simulink model "three_phase_inverter"  (R2014a)
settings: Solver=ode45  StartTime=0.0  StopTime=0.06  MaxStep=0.001  RelTol=1e-3
libraries: powerlib x33
settings Model: Creator=User  LastModifiedBy=User

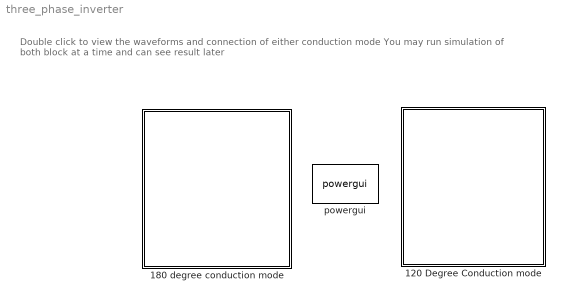
== system three_phase_inverter ==
  note: Double click to view the waveforms and connection of either conduction mode
      | You may run simulation of both block at a time and can see result later
  120 Degree Conduction mode : Subsystem
      mask Display: fprintf('120 degree \n conduction mode')
  180 degree conduction mode : Subsystem
      mask Display: fprintf('180 degree \n conduction mode')
  powergui : powerlib/powergui  Priority=1  SimulationMode=Continuous  SolverType=Tustin  SampleTime=50e-6  frequency=60  SPID=off  DisableSnubberDevices=off  DisableRonSwitches=off  DisableVfSwitches=off  SwTol=0  Interpol=off  DisplayEquations=off  Ts=0  methode=off  frequencyindice=0  Pbase=100e6  ErrMax=1e-4  Iterations=50  UnitsV=kV  UnitsW=MW  FunctionMessages=off  echomessages=off  HookPort=off  EnableUseOfTLC=off  x0status=blocks  RestoreLinks=warning  ResistiveCurrentMeasurement=off  Frange=[0:2:500]  Ylog=off  Xlog=on  ShowGrid=off  save=off  variable=ZData  structure=0  ZoomFFT=off  StartTime=0.0  cycles=1  DisplayStyle=1  fundamental=60  FreqAxis=off  MaxFrequency=1000  frequencyindicesteady=1  RmsSteady=1  display=off

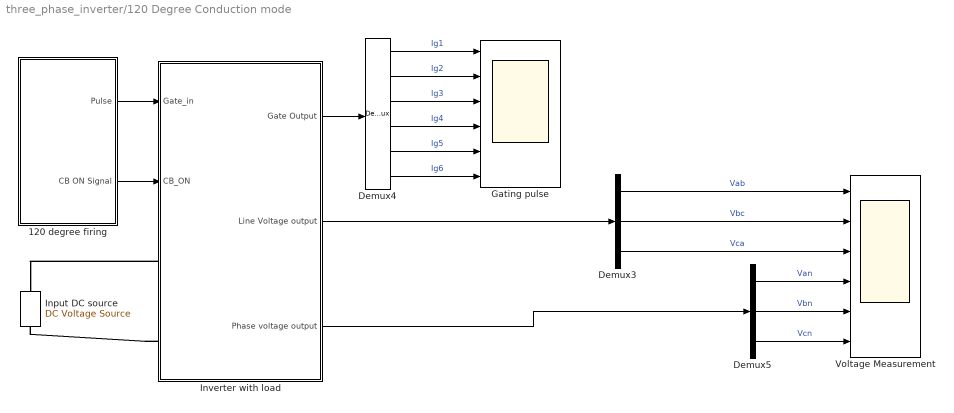
== system three_phase_inverter/120 Degree Conduction mode ==
  120 degree firing : Subsystem  mask{f=50, t=0}
      mask prompts: f "Enter required output frequency"; t "Enter Inverter On time in seconds"
  Demux3 : Demux  Outputs=3
  Demux4 : Demux  Outputs=6
  Demux5 : Demux  Outputs=3
  Gating pulse : Scope  NumInputPorts=6
      settings: ShowLegends=on  YMin=-5~-5~-5~-5~-5~-5  YMax=5~5~5~5~5~5  SaveName=ScopeData2
  Input DC source : powerlib/Electrical Sources/DC Voltage Source  Amplitude=400  Measurements=None
  Inverter with load : Subsystem
  Voltage Measurement : Scope  NumInputPorts=6
      settings: ShowLegends=on  YMin=-5~-5~-5~-5~-5~-5  YMax=5~5~5~5~5~5  SaveName=ScopeData3
  wires:
  Demux4/6 -> Gating pulse/6  "Ig6"
  Inverter with load/2(Line Voltage output) -> Demux3/1
  Demux4/5 -> Gating pulse/5  "Ig5"
  Demux4/2 -> Gating pulse/2  "Ig2"
  Demux3/1 -> Voltage Measurement/1  "Vab"
  120 degree firing/2(CB ON Signal) -> Inverter with load/2(CB_ON)
  Demux4/1 -> Gating pulse/1  "Ig1"
  Demux5/2 -> Voltage Measurement/5  "Vbn"
  Demux4/3 -> Gating pulse/3  "Ig3"
  Demux5/3 -> Voltage Measurement/6  "Vcn"
  Demux5/1 -> Voltage Measurement/4  "Van"
  Demux3/2 -> Voltage Measurement/2  "Vbc"
  Inverter with load/1(Gate Output) -> Demux4/1
  120 degree firing/1(Pulse) -> Inverter with load/1(Gate_in)
  Demux3/3 -> Voltage Measurement/3  "Vca"
  Demux4/4 -> Gating pulse/4  "Ig4"
  Inverter with load/3(Phase voltage output) -> Demux5/1
  connections:
  Inverter with load/LConn1 -- Input DC source/RConn1
  Inverter with load/LConn2 -- Input DC source/LConn1

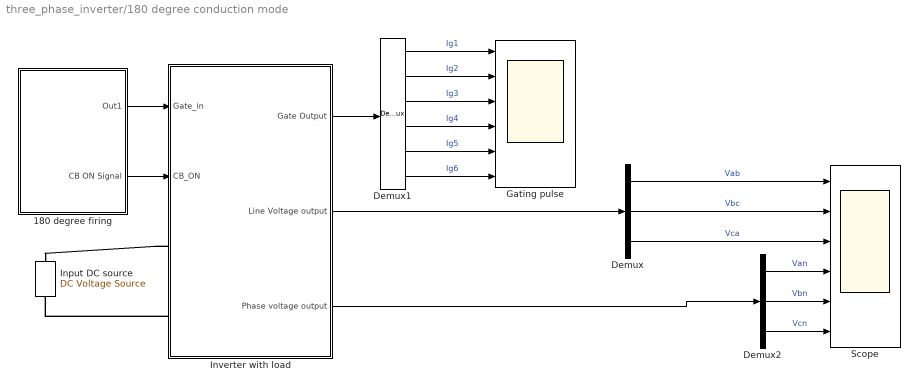
== system three_phase_inverter/180 degree conduction mode ==
  180 degree firing : Subsystem  mask{f=50, t=0}
      mask prompts: f "Enter required output frequency"; t "Enter time to turn ON circuit Breaker in seconds"
  Demux : Demux  Outputs=3
  Demux1 : Demux  Outputs=6
  Demux2 : Demux  Outputs=3
  Gating pulse : Scope  NumInputPorts=6
      settings: ShowLegends=on  YMin=-5~-5~-5~-5~-5~-5  YMax=5~5~5~5~5~5
  Input DC source : powerlib/Electrical Sources/DC Voltage Source  Amplitude=400  Measurements=None
  Inverter with load : Subsystem
  Scope : Scope  NumInputPorts=6
      settings: ShowLegends=on  YMin=-5~-5~-5~-5~-5~-5  YMax=5~5~5~5~5~5
  wires:
  Demux/1 -> Scope/1  "Vab"
  Demux/2 -> Scope/2  "Vbc"
  Demux2/1 -> Scope/4  "Van"
  Demux2/2 -> Scope/5  "Vbn"
  Demux1/4 -> Gating pulse/4  "Ig4"
  Inverter with load/3(Phase voltage output) -> Demux2/1
  Demux1/3 -> Gating pulse/3  "Ig3"
  180 degree firing/1(Out1) -> Inverter with load/1(Gate_in)
  Demux1/6 -> Gating pulse/6  "Ig6"
  Demux1/2 -> Gating pulse/2  "Ig2"
  Demux/3 -> Scope/3  "Vca"
  Demux1/5 -> Gating pulse/5  "Ig5"
  Demux1/1 -> Gating pulse/1  "Ig1"
  Demux2/3 -> Scope/6  "Vcn"
  Inverter with load/1(Gate Output) -> Demux1/1
  Inverter with load/2(Line Voltage output) -> Demux/1
  180 degree firing/2(CB ON Signal) -> Inverter with load/2(CB_ON)
  connections:
  Inverter with load/LConn2 -- Input DC source/LConn1
  Inverter with load/LConn1 -- Input DC source/RConn1

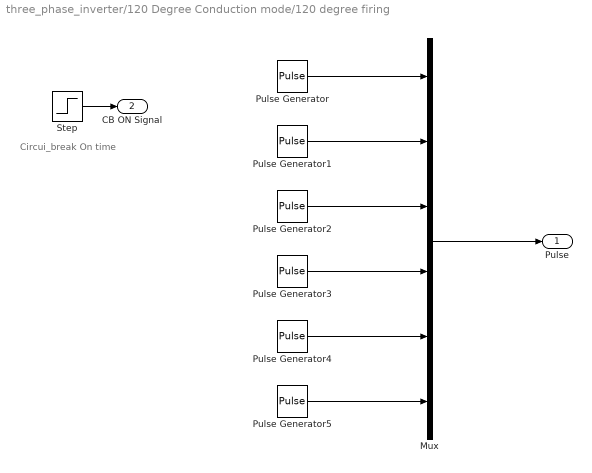
== system three_phase_inverter/120 Degree Conduction mode/120 degree firing ==
  note: Circui_break On time
  Mux : Mux  Inputs=6
  Pulse Generator : DiscretePulseGenerator  PulseType=Time based  Amplitude=5  Period=1/f  PulseWidth=(120/360)*100
  Pulse Generator1 : DiscretePulseGenerator  PulseType=Time based  Amplitude=5  Period=1/f  PulseWidth=(120/360)*100  PhaseDelay=(0.01*60/180)
  Pulse Generator2 : DiscretePulseGenerator  PulseType=Time based  Amplitude=5  Period=1/f  PulseWidth=(120/360)*100  PhaseDelay=0.01*120/180
  Pulse Generator3 : DiscretePulseGenerator  PulseType=Time based  Amplitude=5  Period=1/f  PulseWidth=(120/360)*100  PhaseDelay=0.01
  Pulse Generator4 : DiscretePulseGenerator  PulseType=Time based  Amplitude=5  Period=1/f  PulseWidth=(120/360)*100  PhaseDelay=0.01*240/180
  Pulse Generator5 : DiscretePulseGenerator  PulseType=Time based  Amplitude=5  Period=1/f  PulseWidth=(120/360)*100  PhaseDelay=-0.01*60/180
  Step : Step  Time=t  SampleTime=0
  Pulse : Outport
  CB ON Signal : Outport  Port=2
  wires:
  Pulse Generator/1 -> Mux/1
  Mux/1 -> Pulse/1
  Pulse Generator2/1 -> Mux/3
  Pulse Generator1/1 -> Mux/2
  Pulse Generator3/1 -> Mux/4
  Pulse Generator4/1 -> Mux/5
  Pulse Generator5/1 -> Mux/6
  Step/1 -> CB ON Signal/1

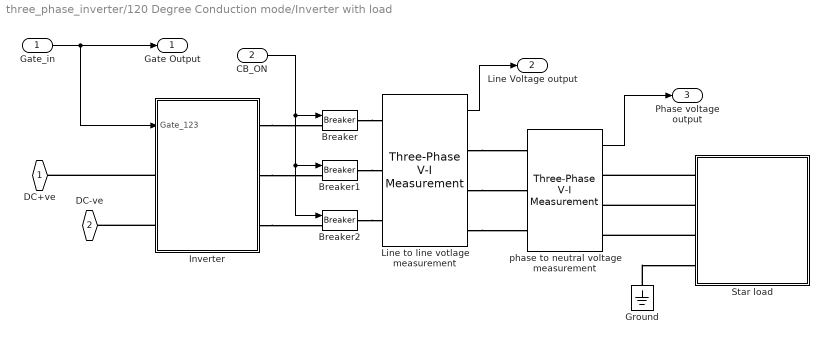
== system three_phase_inverter/120 Degree Conduction mode/Inverter with load ==
  Gate_in : Inport
  CB_ON : Inport  Port=2
  Breaker : powerlib/Elements/Breaker  InitialState=0  SwitchingTimes="[1/60  5/60]"  External=on  BreakerResistance=0.01  SnubberResistance=1e6  SnubberCapacitance=inf  Measurements=None  MoreParameters=on  NoBreakLoop=off
  Breaker1 : powerlib/Elements/Breaker  InitialState=0  SwitchingTimes="[1/60  5/60]"  External=on  BreakerResistance=0.01  SnubberResistance=1e6  SnubberCapacitance=inf  Measurements=None  MoreParameters=on  NoBreakLoop=off
  Breaker2 : powerlib/Elements/Breaker  InitialState=0  SwitchingTimes="[1/60  5/60]"  External=on  BreakerResistance=0.01  SnubberResistance=1e6  SnubberCapacitance=inf  Measurements=None  MoreParameters=on  NoBreakLoop=off
  Ground : powerlib/Elements/Ground  LConnTagsString=a
  Inverter : Subsystem
  Line to line votlage measurement : powerlib/Measurements/Three-Phase V-I Measurement  VoltageMeasurement=phase-to-phase  SetLabelV=off  LabelV=Vabc  Vpu=off  VpuLL=off  CurrentMeasurement=no  SetLabelI=off  LabelI=Iabc  Ipu=off  Pbase=100e6  Vbase=500e3  OutputType=Complex  PhasorSimulation=off  PSBequivalent=0
  Star load : Subsystem
  phase to neutral voltage measurement : powerlib/Measurements/Three-Phase V-I Measurement  VoltageMeasurement=phase-to-ground  SetLabelV=off  LabelV=Vabc  Vpu=off  VpuLL=off  CurrentMeasurement=no  SetLabelI=off  LabelI=Iabc  Ipu=off  Pbase=100e6  Vbase=500e3  OutputType=Complex  PhasorSimulation=off  PSBequivalent=0
  DC+ve : PMIOPort  Port=1  Side=Left
  DC-ve : PMIOPort  Port=2  Side=Left
  Gate Output : Outport
  Line Voltage output : Outport  Port=2
  Phase voltage output : Outport  Port=3
  wires:
  phase to neutral voltage measurement/1 -> Phase voltage output/1
  Line to line votlage measurement/1 -> Line Voltage output/1
  Gate_in/1 -> Gate Output/1, Inverter/1(Gate_123)
  CB_ON/1 -> Breaker2/1, Breaker1/1, Breaker/1
  connections:
  Ground/LConn1 -- Star load/LConn4
  Star load/LConn2 -- phase to neutral voltage measurement/RConn2
  Star load/LConn1 -- phase to neutral voltage measurement/RConn1
  Line to line votlage measurement/RConn3 -- phase to neutral voltage measurement/LConn3
  Line to line votlage measurement/RConn2 -- phase to neutral voltage measurement/LConn2
  Inverter/LConn2 -- DC-ve/RConn1
  Line to line votlage measurement/RConn1 -- phase to neutral voltage measurement/LConn1
  Inverter/LConn1 -- DC+ve/RConn1
  Star load/LConn3 -- phase to neutral voltage measurement/RConn3
  Inverter/RConn1 -- Breaker/LConn1
  Breaker/RConn1 -- Line to line votlage measurement/LConn1
  Inverter/RConn3 -- Breaker2/LConn1
  Inverter/RConn2 -- Breaker1/LConn1
  Breaker1/RConn1 -- Line to line votlage measurement/LConn2
  Breaker2/RConn1 -- Line to line votlage measurement/LConn3

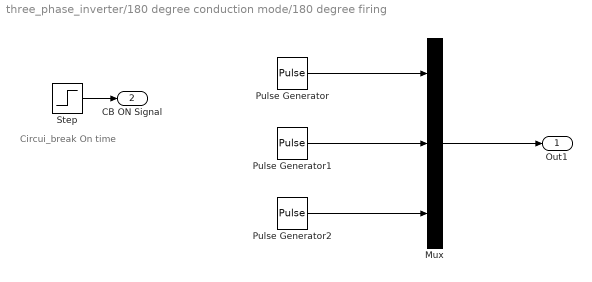
== system three_phase_inverter/180 degree conduction mode/180 degree firing ==
  note: Circui_break On time
  Mux : Mux  Inputs=3
  Pulse Generator : DiscretePulseGenerator  PulseType=Time based  Amplitude=5  Period=1/f  PulseWidth=50
  Pulse Generator1 : DiscretePulseGenerator  PulseType=Time based  Amplitude=5  Period=1/f  PulseWidth=50  PhaseDelay=(0.01*60/180)
  Pulse Generator2 : DiscretePulseGenerator  PulseType=Time based  Amplitude=5  Period=1/f  PulseWidth=50  PhaseDelay=0.01*120/180
  Step : Step  Time=t  SampleTime=0
  Out1 : Outport
  CB ON Signal : Outport  Port=2
  wires:
  Pulse Generator1/1 -> Mux/2
  Pulse Generator2/1 -> Mux/3
  Mux/1 -> Out1/1
  Pulse Generator/1 -> Mux/1
  Step/1 -> CB ON Signal/1

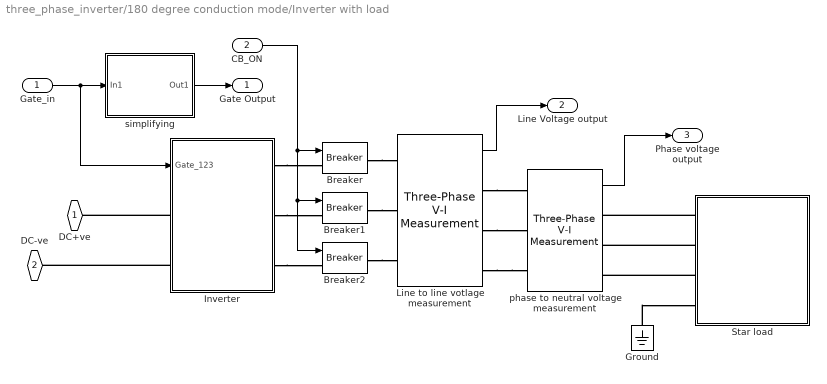
== system three_phase_inverter/180 degree conduction mode/Inverter with load ==
  Gate_in : Inport
  CB_ON : Inport  Port=2
  Breaker : powerlib/Elements/Breaker  InitialState=0  SwitchingTimes="[1/60  5/60]"  External=on  BreakerResistance=0.01  SnubberResistance=1e6  SnubberCapacitance=inf  Measurements=None  MoreParameters=on  NoBreakLoop=off
  Breaker1 : powerlib/Elements/Breaker  InitialState=0  SwitchingTimes="[1/60  5/60]"  External=on  BreakerResistance=0.01  SnubberResistance=1e6  SnubberCapacitance=inf  Measurements=None  MoreParameters=on  NoBreakLoop=off
  Breaker2 : powerlib/Elements/Breaker  InitialState=0  SwitchingTimes="[1/60  5/60]"  External=on  BreakerResistance=0.01  SnubberResistance=1e6  SnubberCapacitance=inf  Measurements=None  MoreParameters=on  NoBreakLoop=off
  Ground : powerlib/Elements/Ground  LConnTagsString=a
  Inverter : Subsystem
  Line to line votlage measurement : powerlib/Measurements/Three-Phase V-I Measurement  VoltageMeasurement=phase-to-phase  SetLabelV=off  LabelV=Vabc  Vpu=off  VpuLL=off  CurrentMeasurement=no  SetLabelI=off  LabelI=Iabc  Ipu=off  Pbase=100e6  Vbase=500e3  OutputType=Complex  PhasorSimulation=off  PSBequivalent=0
  Star load : Subsystem
  phase to neutral voltage measurement : powerlib/Measurements/Three-Phase V-I Measurement  VoltageMeasurement=phase-to-ground  SetLabelV=off  LabelV=Vabc  Vpu=off  VpuLL=off  CurrentMeasurement=no  SetLabelI=off  LabelI=Iabc  Ipu=off  Pbase=100e6  Vbase=500e3  OutputType=Complex  PhasorSimulation=off  PSBequivalent=0
  simplifying : Subsystem
  DC+ve : PMIOPort  Port=1  Side=Left
  DC-ve : PMIOPort  Port=2  Side=Left
  Gate Output : Outport
  Line Voltage output : Outport  Port=2
  Phase voltage output : Outport  Port=3
  wires:
  simplifying/1(Out1) -> Gate Output/1
  Line to line votlage measurement/1 -> Line Voltage output/1
  Gate_in/1 -> Inverter/1(Gate_123), simplifying/1(In1)
  phase to neutral voltage measurement/1 -> Phase voltage output/1
  CB_ON/1 -> Breaker2/1, Breaker1/1, Breaker/1
  connections:
  Star load/LConn3 -- phase to neutral voltage measurement/RConn3
  Inverter/LConn1 -- DC+ve/RConn1
  Line to line votlage measurement/RConn1 -- phase to neutral voltage measurement/LConn1
  Inverter/LConn2 -- DC-ve/RConn1
  Line to line votlage measurement/RConn2 -- phase to neutral voltage measurement/LConn2
  Line to line votlage measurement/RConn3 -- phase to neutral voltage measurement/LConn3
  Star load/LConn1 -- phase to neutral voltage measurement/RConn1
  Star load/LConn2 -- phase to neutral voltage measurement/RConn2
  Ground/LConn1 -- Star load/LConn4
  Inverter/RConn1 -- Breaker/LConn1
  Inverter/RConn2 -- Breaker1/LConn1
  Inverter/RConn3 -- Breaker2/LConn1
  Breaker/RConn1 -- Line to line votlage measurement/LConn1
  Breaker1/RConn1 -- Line to line votlage measurement/LConn2
  Breaker2/RConn1 -- Line to line votlage measurement/LConn3

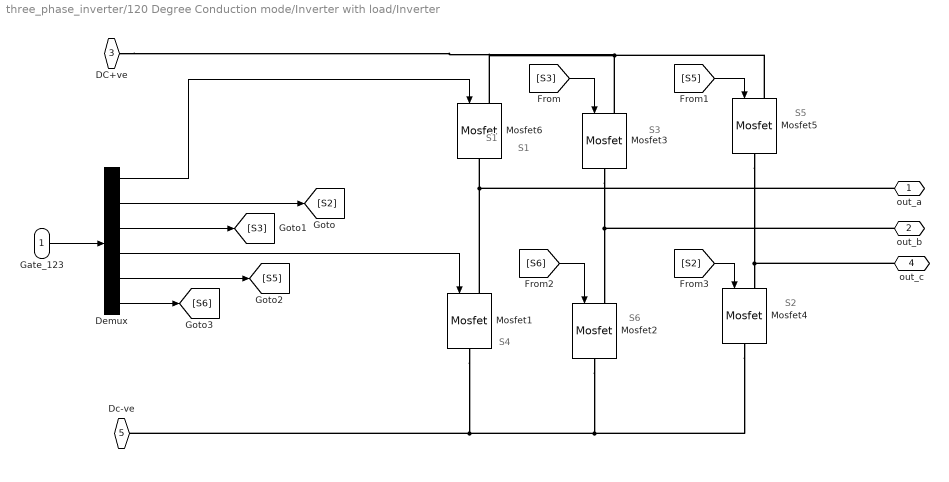
== system three_phase_inverter/120 Degree Conduction mode/Inverter with load/Inverter ==
  note: S1
  note: S3
  note: S5
  note: S2
  note: S4
  note: S6
  note: S1
  Gate_123 : Inport
  Demux : Demux  Outputs=6
  Mosfet{1..6} (6 alike) : powerlib/Power Electronics/Mosfet  Ron=0.1  Lon=0  Rd=0.01  Vfd=0  IC=0  Rs=1e5  Cs=inf  Measurements=off
  out_a : PMIOPort  Port=1  Side=Right
  out_b : PMIOPort  Port=2  Side=Right
  DC+ve : PMIOPort  Port=3  Side=Left
  out_c : PMIOPort  Port=4  Side=Right
  Dc-ve : PMIOPort  Port=5  Side=Left
  wires:
  [S5] -> Mosfet5/1
  [S2] -> Mosfet4/1
  [S6] -> Mosfet2/1
  [S3] -> Mosfet3/1
  Demux/1 -> Mosfet6/1
  Gate_123/1 -> Demux/1
  Demux/2 -> [S2]
  Demux/3 -> [S3]
  Demux/4 -> Mosfet1/1
  Demux/5 -> [S5]
  Demux/6 -> [S6]
  connections:
  out_c/RConn1 -- Mosfet5/RConn1 -- Mosfet4/LConn1
  out_b/RConn1 -- Mosfet2/LConn1 -- Mosfet3/RConn1
  Mosfet4/RConn1 -- Mosfet2/RConn1 -- Mosfet1/RConn1 -- Dc-ve/RConn1
  Mosfet5/LConn1 -- Mosfet6/LConn1 -- DC+ve/RConn1 -- Mosfet3/LConn1
  out_a/RConn1 -- Mosfet1/LConn1 -- Mosfet6/RConn1

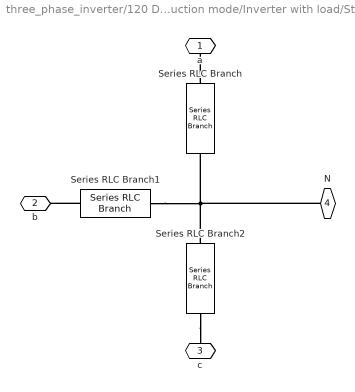
== system three_phase_inverter/120 Degree Conduction mode/Inverter with load/Star load ==
  Series RLC Branch : powerlib/Elements/Series RLC Branch  LConnTagsString=__new0  RConnTagsString=__new0  BranchType=R  Resistance=10  Inductance=1e-3  SetiL0=off  InitialCurrent=0  Capacitance=1e-6  Setx0=off  InitialVoltage=0  Measurements=None
  Series RLC Branch1 : powerlib/Elements/Series RLC Branch  LConnTagsString=__new0  RConnTagsString=__new0  BranchType=R  Resistance=10  Inductance=1e-3  SetiL0=off  InitialCurrent=0  Capacitance=1e-6  Setx0=off  InitialVoltage=0  Measurements=None
  Series RLC Branch2 : powerlib/Elements/Series RLC Branch  LConnTagsString=__new0  RConnTagsString=__new0  BranchType=R  Resistance=10  Inductance=1e-3  SetiL0=off  InitialCurrent=0  Capacitance=1e-6  Setx0=off  InitialVoltage=0  Measurements=None
  a : PMIOPort  Port=1  Side=Left
  b : PMIOPort  Port=2  Side=Left
  c : PMIOPort  Port=3  Side=Left
  N : PMIOPort  Port=4  Side=Left
  connections:
  Series RLC Branch/LConn1 -- a/RConn1
  Series RLC Branch1/RConn1 -- b/RConn1
  Series RLC Branch2/RConn1 -- c/RConn1
  Series RLC Branch2/LConn1 -- N/RConn1 -- Series RLC Branch/RConn1 -- Series RLC Branch1/LConn1

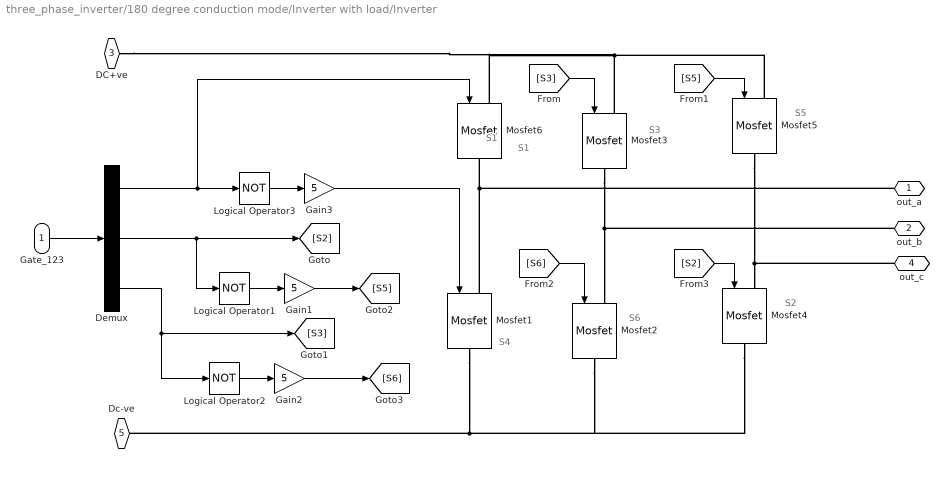
== system three_phase_inverter/180 degree conduction mode/Inverter with load/Inverter ==
  note: S1
  note: S6
  note: S4
  note: S2
  note: S5
  note: S3
  note: S1
  Gate_123 : Inport
  Demux : Demux  Outputs=3
  Gain1 : Gain  Gain=5
  Gain2 : Gain  Gain=5
  Gain3 : Gain  Gain=5
  Logical Operator1 : Logic  Operator=NOT  AllPortsSameDT=off  OutDataTypeStr=boolean
  Logical Operator2 : Logic  Operator=NOT  AllPortsSameDT=off  OutDataTypeStr=boolean
  Logical Operator3 : Logic  Operator=NOT  AllPortsSameDT=off  OutDataTypeStr=boolean
  Mosfet{1..6} (6 alike) : powerlib/Power Electronics/Mosfet  Ron=0.1  Lon=0  Rd=0.01  Vfd=0  IC=0  Rs=1e5  Cs=inf  Measurements=off
  out_a : PMIOPort  Port=1  Side=Right
  out_b : PMIOPort  Port=2  Side=Right
  DC+ve : PMIOPort  Port=3  Side=Left
  out_c : PMIOPort  Port=4  Side=Right
  Dc-ve : PMIOPort  Port=5  Side=Left
  wires:
  Gate_123/1 -> Demux/1
  Logical Operator3/1 -> Gain3/1
  Demux/1 -> Logical Operator3/1, Mosfet6/1
  Gain3/1 -> Mosfet1/1
  Demux/2 -> Logical Operator1/1, [S2]
  Demux/3 -> [S3], Logical Operator2/1
  Logical Operator1/1 -> Gain1/1
  Logical Operator2/1 -> Gain2/1
  Gain1/1 -> [S5]
  Gain2/1 -> [S6]
  [S3] -> Mosfet3/1
  [S6] -> Mosfet2/1
  [S2] -> Mosfet4/1
  [S5] -> Mosfet5/1
  connections:
  Mosfet1/LConn1 -- out_a/RConn1 -- Mosfet6/RConn1
  DC+ve/RConn1 -- Mosfet6/LConn1 -- Mosfet5/LConn1 -- Mosfet3/LConn1
  Mosfet1/RConn1 -- Mosfet4/RConn1 -- Mosfet2/RConn1 -- Dc-ve/RConn1
  Mosfet3/RConn1 -- out_b/RConn1 -- Mosfet2/LConn1
  Mosfet5/RConn1 -- out_c/RConn1 -- Mosfet4/LConn1

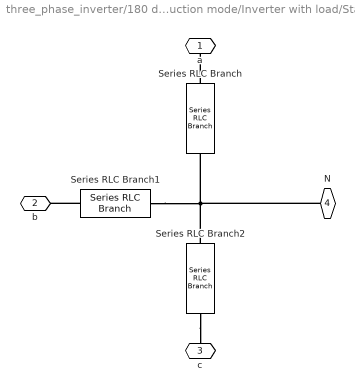
== system three_phase_inverter/180 degree conduction mode/Inverter with load/Star load ==
  Series RLC Branch : powerlib/Elements/Series RLC Branch  LConnTagsString=__new0  RConnTagsString=__new0  BranchType=R  Resistance=10  Inductance=1e-3  SetiL0=off  InitialCurrent=0  Capacitance=1e-6  Setx0=off  InitialVoltage=0  Measurements=None
  Series RLC Branch1 : powerlib/Elements/Series RLC Branch  LConnTagsString=__new0  RConnTagsString=__new0  BranchType=R  Resistance=10  Inductance=1e-3  SetiL0=off  InitialCurrent=0  Capacitance=1e-6  Setx0=off  InitialVoltage=0  Measurements=None
  Series RLC Branch2 : powerlib/Elements/Series RLC Branch  LConnTagsString=__new0  RConnTagsString=__new0  BranchType=R  Resistance=10  Inductance=1e-3  SetiL0=off  InitialCurrent=0  Capacitance=1e-6  Setx0=off  InitialVoltage=0  Measurements=None
  a : PMIOPort  Port=1  Side=Left
  b : PMIOPort  Port=2  Side=Left
  c : PMIOPort  Port=3  Side=Left
  N : PMIOPort  Port=4  Side=Left
  connections:
  Series RLC Branch1/LConn1 -- Series RLC Branch/RConn1 -- N/RConn1 -- Series RLC Branch2/LConn1
  Series RLC Branch2/RConn1 -- c/RConn1
  Series RLC Branch1/RConn1 -- b/RConn1
  Series RLC Branch/LConn1 -- a/RConn1

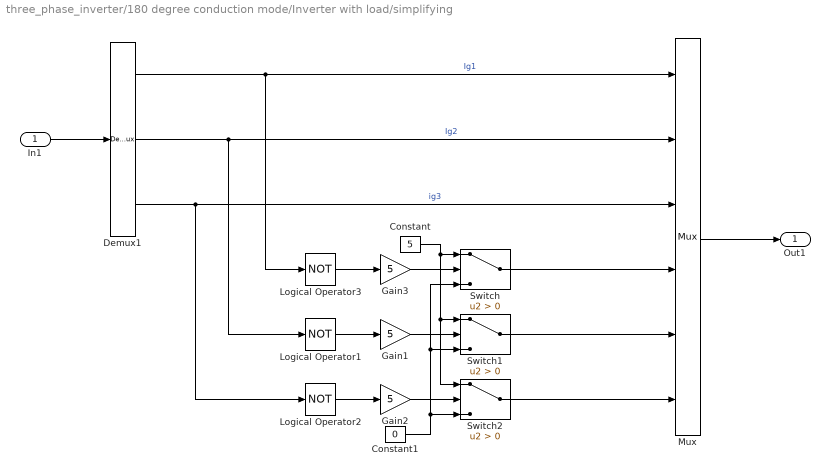
== system three_phase_inverter/180 degree conduction mode/Inverter with load/simplifying ==
  In1 : Inport
  Constant : Constant  Value=5
  Constant1 : Constant  Value=0
  Demux1 : Demux  Outputs=3
  Gain1 : Gain  Gain=5
  Gain2 : Gain  Gain=5
  Gain3 : Gain  Gain=5
  Logical Operator1 : Logic  Operator=NOT  AllPortsSameDT=off  OutDataTypeStr=boolean
  Logical Operator2 : Logic  Operator=NOT  AllPortsSameDT=off  OutDataTypeStr=boolean
  Logical Operator3 : Logic  Operator=NOT  AllPortsSameDT=off  OutDataTypeStr=boolean
  Mux : Mux  Inputs=6
  Switch : Switch  Criteria=u2 > Threshold
  Switch1 : Switch  Criteria=u2 > Threshold
  Switch2 : Switch  Criteria=u2 > Threshold
  Out1 : Outport
  wires:
  Mux/1 -> Out1/1
  In1/1 -> Demux1/1
  Demux1/3 -> Logical Operator2/1, Mux/3  "ig3"
  Demux1/2 -> Logical Operator1/1, Mux/2  "Ig2"
  Demux1/1 -> Logical Operator3/1, Mux/1  "Ig1"
  Logical Operator3/1 -> Gain3/1
  Logical Operator1/1 -> Gain1/1
  Logical Operator2/1 -> Gain2/1
  Gain3/1 -> Switch/2
  Gain1/1 -> Switch1/2
  Gain2/1 -> Switch2/2
  Constant/1 -> Switch2/1, Switch1/1, Switch/1
  Constant1/1 -> Switch/3, Switch1/3, Switch2/3
  Switch/1 -> Mux/4
  Switch1/1 -> Mux/5
  Switch2/1 -> Mux/6
